simulink model "Delay"  (R2021b)
settings: Solver=ode1  StartTime=0.0  StopTime=inf  FixedStep=0.001  RelTol=1e-3
undefined symbols (not defined in the file): delayTimeCarToDamper
settings Model: Creator=jalfonso  LastModifiedBy=au602135
settings SolverCC: AlgebraicLoopSolver=TrustRegion
settings DataIOCC: ReturnWorkspaceOutputs=off
settings DebuggingCC: SFMachineParentedDataDiag=warning  ArithmeticOperatorsInVariantConditions=warning
settings SFSimCC: SimUseLocalCustomCode=off  CustomCodeUndefinedFunction=UseInterfaceOnly
settings RTWCC: RTWUseLocalCustomCode=off
settings CodeAppCC: StateflowObjectComments=on

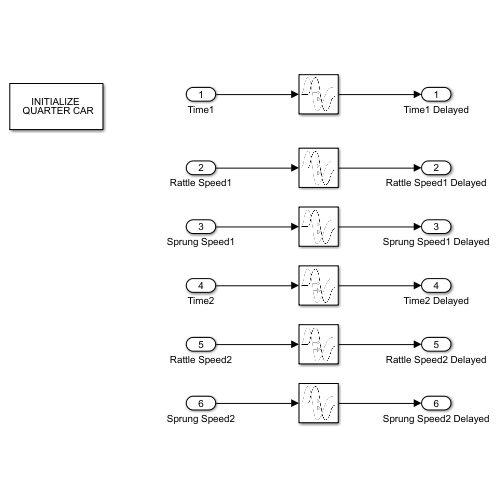
[thumbnail: Simulink's stored preview of the top-level diagram]
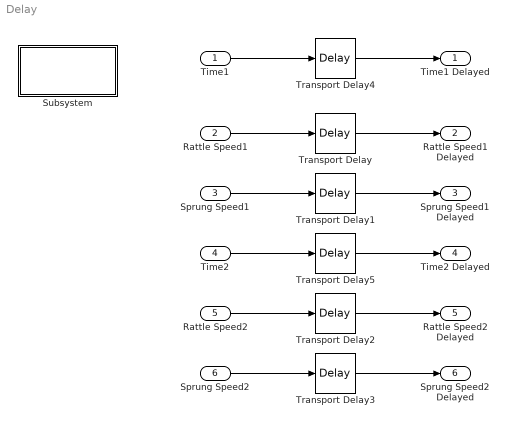
== system Delay ==
  Time1 : Inport
  Rattle Speed1 : Inport  Port=2
  Sprung Speed1 : Inport  Port=3
  Time2 : Inport  Port=4
  Rattle Speed2 : Inport  Port=5
  Sprung Speed2 : Inport  Port=6
  Subsystem : Subsystem
      settings: OpenFcn=|
      | k_tire = 225400;  %200000 in literature
      | c_tire = 100;        % Estimated. In literatures 6N
      | k_susp =  25000;  % 15000 in literature
      | c_susp = 400;       %1429 Ns/m in literature
      | g = 0 % 9.8; Removed to avoid initialization problems
      | m_unsprung = 66;
      | m_sprung = 449.25;
      | X_sprung0  = .5;
      | X_unsprung0  = .1;
      | delayTimeCarToDamper =  0.002;
      | %InitQuarterCarCompensatorScript;
      | %Amplitude =.01;
      mask Display: disp('INITIALIZE \n QUARTER CAR')
  Transport Delay{,1..5} (6 alike) : TransportDelay  DelayTime=delayTimeCarToDamper
  Time1 Delayed : Outport
  Rattle Speed1 Delayed : Outport  Port=2
  Sprung Speed1 Delayed : Outport  Port=3
  Time2 Delayed : Outport  Port=4
  Rattle Speed2 Delayed : Outport  Port=5
  Sprung Speed2 Delayed : Outport  Port=6
  wires:
  Transport Delay/1 -> Rattle Speed1 Delayed/1
  Transport Delay1/1 -> Sprung Speed1 Delayed/1
  Transport Delay2/1 -> Rattle Speed2 Delayed/1
  Transport Delay3/1 -> Sprung Speed2 Delayed/1
  Transport Delay5/1 -> Time2 Delayed/1
  Transport Delay4/1 -> Time1 Delayed/1
  Time1/1 -> Transport Delay4/1
  Rattle Speed1/1 -> Transport Delay/1
  Sprung Speed1/1 -> Transport Delay1/1
  Time2/1 -> Transport Delay5/1
  Rattle Speed2/1 -> Transport Delay2/1
  Sprung Speed2/1 -> Transport Delay3/1

== system Delay/Subsystem ==
